simulink model "LAB_07_SIM_1"  (R2022b)
settings: Solver=ode4  StartTime=0.0  StopTime=10000  FixedStep=0.1  RelTol=1e-3
values from neighbouring files (symbols this model uses):
  a = 16371e+3    (= 16371000)    [lab_07_MAT.m]
  A0 = diag([1 1 1])    [LAB_04_17_OCT_MAT_KIN.m]    (also in LAB_05_24_OCT_MAT_KIN_COSDIR.m; LAB_06.m = A_target_fun(0); core_attitude_test.m = eye(3,3); lab_07_MAT.m)
  A_B1 = 2e-2    (= 0.02)    [lab_07_MAT.m]
  A_B2 = 6e-2    (= 0.06)    [lab_07_MAT.m]
  A_B3 = 2e-2    (= 0.02)    [lab_07_MAT.m]
  A_B4 = 6e-2    (= 0.06)    [lab_07_MAT.m]
  A_B5 = 3e-2    (= 0.03)    [lab_07_MAT.m]
  A_B6 = 3e-2    (= 0.03)    [lab_07_MAT.m]
  A_P1 = 12e-2    (= 0.12)    [lab_07_MAT.m]
  A_P2 = 12e-2    (= 0.12)    [lab_07_MAT.m]
  A_P3 = 12e-2    (= 0.12)    [lab_07_MAT.m]
  A_P4 = 12e-2    (= 0.12)    [lab_07_MAT.m]
  ang = deg2rad(11.5)    [lab_07_MAT.m]
  e = 0    [lab_07_MAT.m]
  g_1_0 = -29404.8    [lab_07_MAT.m]
  g_1_1 = -1450.9    [lab_07_MAT.m]
  h_1_1 = 4652.5    [lab_07_MAT.m]
  I = [Ix 0 0 ... (first row only)    [LAB_03_3_OCT_MAT_EUL_2_VERIFICATION.m]    (also in LAB_03_3_OCT_MAT_EUL_DOUBLESPIN.m = diag([Ix, Iy, Iz]); LAB_03_3_OCT_MAT_EUL_SPINAXIS.m = diag([Ix, Iy, Iz]); LAB_03_3_OCT_MAT_EUL_VECT.m; LAB_04_17_OCT_MAT_KIN.m)
  i = char('pippo')    [LAB_01_19_SEPT.m]    (also in lab_07_MAT.m = 0.1)
  j_B = [0.01; 0.05; 0.01]    [lab_07_MAT.m]
  N_B1 = [1,0,0]'    [lab_07_MAT.m]
  N_B2 = [0,1,0]'    [lab_07_MAT.m]
  N_B3 = [-1,0,0]'    [lab_07_MAT.m]
  N_B4 = [0,-1,0]'    [lab_07_MAT.m]
  N_B5 = [0,0,1]'    [lab_07_MAT.m]
  N_B6 = [0,0,-1]    [lab_07_MAT.m]
  N_P1 = [0,0,1]    [lab_07_MAT.m]
  N_P2 = [0,0,-1]    [lab_07_MAT.m]
  N_P3 = [0,0,1]    [lab_07_MAT.m]
  N_P4 = [0,0,-1]    [lab_07_MAT.m]
  n_rot = 0.0012    [lab_07_MAT.m]
  n_sun = 2*pi/T    (= 1.99238499086e-07)    [lab_07_MAT.m]
  om_0 = [om_x0, om_y0, om_z0]    [LAB_03_3_OCT_MAT_EUL.m]    (also in LAB_03_3_OCT_MAT_EUL_2_VERIFICATION.m = [om_x0; om_y0; om_z0]; LAB_03_3_OCT_MAT_EUL_DOUBLESPIN.m = [om_x0; om_y0; om_z0]; LAB_03_3_OCT_MAT_EUL_SPINAXIS.m = [om_x0; om_y0; om_z0]; LAB_03_3_OCT_MAT_EUL_VECT.m = [om_x0; om_y0; om_z0])
  P = [Px, Py, Pz]    [LAB_03_3_OCT_MAT_EUL_VECT.m]    (also in lab_07_MAT.m = 4.52666666667e-06)
  R = 6.371e+6 + H    (= 6381000)    [LAB_06.m]    (also in lab_07_MAT.m = 6378000)
  r_B1 = 1e-2*[15,0,0]    [lab_07_MAT.m]
  r_B2 = 1e-2*[0,5,0]    [lab_07_MAT.m]
  r_B3 = 1e-2*[-15,0,0]    [lab_07_MAT.m]
  r_B4 = 1e-2*[0,-5,0]    [lab_07_MAT.m]
  r_B5 = 1e-2*[0,0,10]    [lab_07_MAT.m]
  r_B6 = 1e-2*[0,0,-10]    [lab_07_MAT.m]
  r_P1 = 1e-2*[0,20,10]    [lab_07_MAT.m]
  r_P2 = 1e-2*[0,20,10]    [lab_07_MAT.m]
  r_P3 = 1e-2*[0,-20,10]    [lab_07_MAT.m]
  r_P4 = 1e-2*[0,-20,10]    [lab_07_MAT.m]
  r_sun = 149597870000    [lab_07_MAT.m]
  rho_d = 0.1    [lab_07_MAT.m]
  rho_sB = 0.5    [lab_07_MAT.m]
  rho_sP = 0.5    [lab_07_MAT.m]
  rot_E = 7.29e-5    (= 7.29e-05)    [lab_07_MAT.m]
  theta_0 = 3/2 * pi    (= 4.71238898038)    [lab_07_MAT.m]
libraries: matrix_library x12, sharedutil x1, vrlib x1
settings Model: Creator=maria  LastModifiedBy=maria

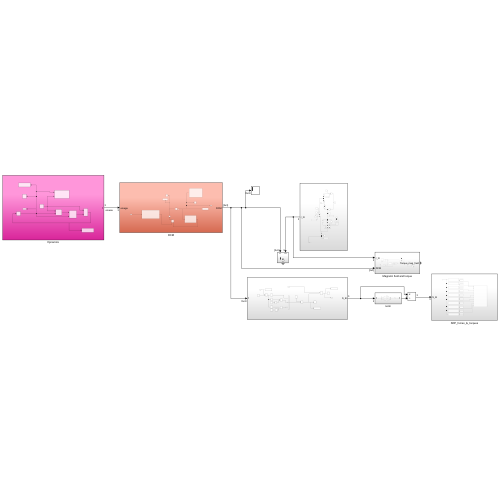
[thumbnail: Simulink's stored preview of the top-level diagram]
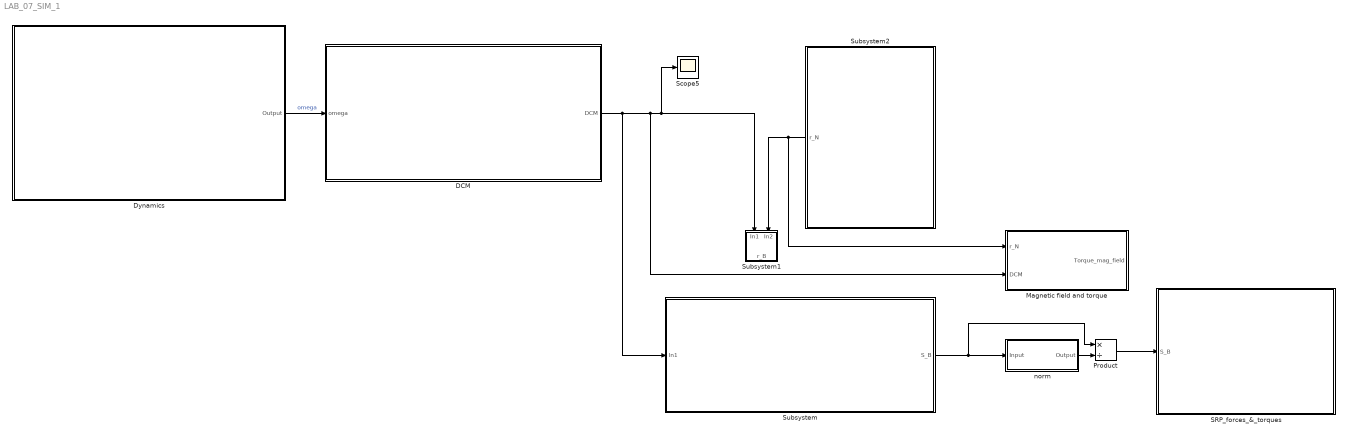
== system LAB_07_SIM_1 ==
  DCM : Subsystem
  Dynamics : Subsystem
  Magnetic field and torque : Subsystem
  Product : Product  Inputs=*/
  SRP_forces_&_torques : Subsystem
  Scope5 : Scope
  Subsystem : Subsystem
  Subsystem1 : Subsystem
  Subsystem2 : Subsystem
  norm : Subsystem
  wires:
  Dynamics/1(Output) -> DCM/1(omega)  "omega"
  DCM/1(DCM) -> Subsystem/1(In1), Magnetic field and torque/2(DCM), Subsystem1/1(In1), Scope5/1
  Subsystem2/1(r_N) -> Magnetic field and torque/1(r_N), Subsystem1/2(In2)
  Subsystem/1(S_B) -> Product/1, norm/1(Input)
  norm/1(Output) -> Product/2
  Product/1 -> SRP_forces_&_torques/1(S_B)

== system LAB_07_SIM_1/DCM ==
  note: A
  omega : Inport
  Determinant Chech fo Validation : Subsystem
  Gain1 : Gain  Gain=-1
  Integrator1 : Integrator  InitialCondition=A0
  Product2 : Product  Multiplication=Matrix(*)
  Scope1 : Scope
  Scope2 : Scope
  Subsystem : Subsystem
  To Workspace2 : ToWorkspace  VariableName=A  SampleTime=-1
  To Workspace3 : ToWorkspace  VariableName=A_dot  SampleTime=-1
  matrix of omega cross prod : Subsystem
  DCM : Outport
  wires:
  Integrator1/1 -> Subsystem/1(A1), Scope2/1, Determinant Chech fo Validation/1(DCM), DCM/1, To Workspace2/1
  matrix of omega cross prod/1(Out1) -> Product2/1
  Product2/1 -> Gain1/1  "A_dot"
  omega/1 -> matrix of omega cross prod/1(om)
  Gain1/1 -> Integrator1/1, To Workspace3/1, Scope1/1
  Subsystem/1(A_orthonormalized1) -> Product2/2

== system LAB_07_SIM_1/Dynamics ==
  Constant : Constant  Value=I
  Cross Product : matrix_library/Cross Product
  Integrator : Integrator  InitialCondition=om_0
  Product : Product  Multiplication=Matrix(*)
  Product1 : Product  Inputs=/*  Multiplication=Matrix(*)
  Scope : Scope
  To Workspace1 : ToWorkspace  VariableName=omega  SampleTime=-1
  To Workspace2 : ToWorkspace  VariableName=omega_dot  SampleTime=-1
  validation : Subsystem
  Output : Outport
  wires:
  Product1/1 -> To Workspace2/1, Integrator/1  "om_dot"
  Integrator/1 -> Product/2, Cross Product/2, validation/1(om), To Workspace1/1, Scope/1, Output/1  "om"
  Cross Product/1 -> Product1/2
  Constant/1 -> Product1/1, Product/1, validation/2(In2)  "I"
  Product/1 -> Cross Product/1

== system LAB_07_SIM_1/Magnetic field and torque ==
  r_N : Inport
  DCM : Inport  Port=2
  Constant : Constant  Value=j_B
  Constant10 : Constant  Value=3
  Constant5 : Constant  Value=R
  Constant9 : Constant  Value=3
  Cross Product : matrix_library/Cross Product
  Dot Product : DotProduct  OutDataTypeStr=Inherit: Inherit via internal rule
  Gain : Gain  Gain=1e-9
  Gain1 : Gain  Gain=3
  MatrixMultiply : Product  Multiplication=Matrix(*)
  Normalize Vector : vrlib/Utilities/Normalize Vector  maxzero=0
  Power : Math  Operator=pow
  Power1 : Math  Operator=pow
  Product3 : Product  Inputs=**/
  Product4 : Product
  Product5 : Product
  Scope : Scope
  Scope1 : Scope
  Scope3 : Scope
  Subsystem : Subsystem
  Sum1 : Sum  Inputs=-+
  To Workspace : ToWorkspace  VariableName=b_N  SampleTime=-1
  To Workspace3 : ToWorkspace  VariableName=Torque_mag_field  SampleTime=-1
  m : Subsystem
  norm1 : Subsystem
  Torque_mag_field : Outport
  wires:
  r_N/1 -> Normalize Vector/1, norm1/1(Input)
  Constant5/1 -> Power/1
  Constant9/1 -> Power/2
  Power/1 -> Product3/2
  Constant10/1 -> Power1/2
  norm1/1(Output) -> Power1/1  "r_norm"
  Power1/1 -> Product3/3
  Product3/1 -> Product4/1
  Dot Product/1 -> Product5/1
  m/1(m) -> Sum1/1, Dot Product/1
  Normalize Vector/1 -> Product5/2, Dot Product/2
  Product5/1 -> Gain1/1
  Sum1/1 -> Product4/2
  Subsystem/1(H0) -> Gain/1
  Product4/1 -> MatrixMultiply/2, To Workspace/1, Scope/1
  MatrixMultiply/1 -> Cross Product/2, Scope3/1, To Workspace3/1  "b_B"
  DCM/1 -> MatrixMultiply/1
  Constant/1 -> Cross Product/1
  Cross Product/1 -> Scope1/1, Torque_mag_field/1
  Gain1/1 -> Sum1/2
  Gain/1 -> Product3/1

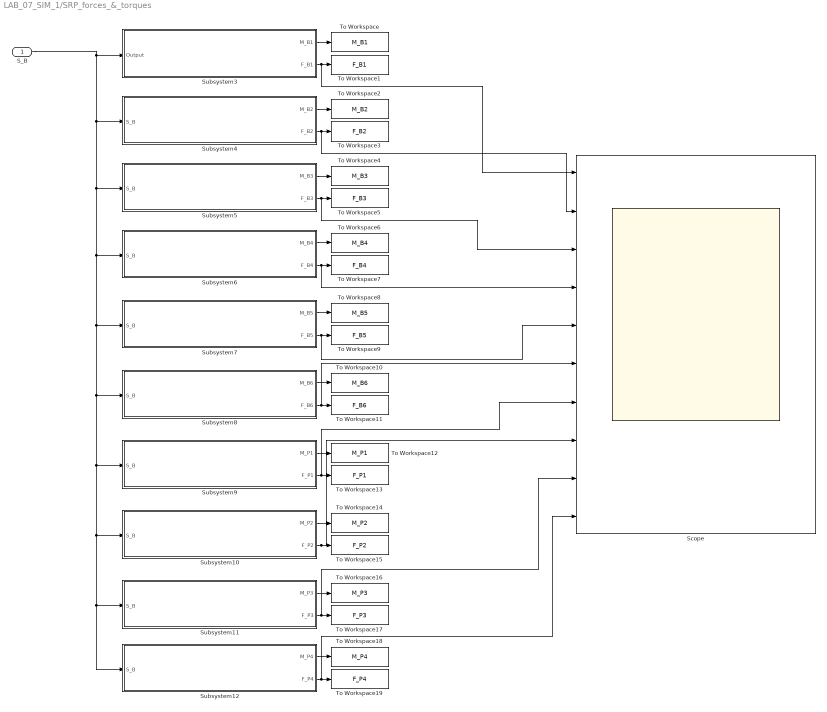
== system LAB_07_SIM_1/SRP_forces_&_torques ==
  S_B : Inport
  Scope : Scope  NumInputPorts=10
  Subsystem10 : Subsystem
  Subsystem11 : Subsystem
  Subsystem12 : Subsystem
  Subsystem3 : Subsystem
  Subsystem4 : Subsystem
  Subsystem5 : Subsystem
  Subsystem6 : Subsystem
  Subsystem7 : Subsystem
  Subsystem8 : Subsystem
  Subsystem9 : Subsystem
  To Workspace : ToWorkspace  VariableName=M_B1  SampleTime=-1
  To Workspace1 : ToWorkspace  VariableName=F_B1  SampleTime=-1
  To Workspace10 : ToWorkspace  VariableName=M_B6  SampleTime=-1
  To Workspace11 : ToWorkspace  VariableName=F_B6  SampleTime=-1
  To Workspace12 : ToWorkspace  VariableName=M_P1  SampleTime=-1
  To Workspace13 : ToWorkspace  VariableName=F_P1  SampleTime=-1
  To Workspace14 : ToWorkspace  VariableName=M_P2  SampleTime=-1
  To Workspace15 : ToWorkspace  VariableName=F_P2  SampleTime=-1
  To Workspace16 : ToWorkspace  VariableName=M_P3  SampleTime=-1
  To Workspace17 : ToWorkspace  VariableName=F_P3  SampleTime=-1
  To Workspace18 : ToWorkspace  VariableName=M_P4  SampleTime=-1
  To Workspace19 : ToWorkspace  VariableName=F_P4  SampleTime=-1
  To Workspace2 : ToWorkspace  VariableName=M_B2  SampleTime=-1
  To Workspace3 : ToWorkspace  VariableName=F_B2  SampleTime=-1
  To Workspace4 : ToWorkspace  VariableName=M_B3  SampleTime=-1
  To Workspace5 : ToWorkspace  VariableName=F_B3  SampleTime=-1
  To Workspace6 : ToWorkspace  VariableName=M_B4  SampleTime=-1
  To Workspace7 : ToWorkspace  VariableName=F_B4  SampleTime=-1
  To Workspace8 : ToWorkspace  VariableName=M_B5  SampleTime=-1
  To Workspace9 : ToWorkspace  VariableName=F_B5  SampleTime=-1
  wires:
  S_B/1 -> Subsystem11/1(S_B), Subsystem12/1(S_B), Subsystem10/1(S_B), Subsystem9/1(S_B), Subsystem8/1(S_B), Subsystem7/1(S_B), Subsystem6/1(S_B), Subsystem5/1(S_B), Subsystem4/1(S_B), Subsystem3/1(Output)
  Subsystem7/2(F_B5) -> Scope/5, To Workspace9/1
  Subsystem12/2(F_P4) -> Scope/10, To Workspace19/1
  Subsystem12/1(M_P4) -> To Workspace18/1
  Subsystem6/1(M_B4) -> To Workspace6/1
  Subsystem7/1(M_B5) -> To Workspace8/1
  Subsystem8/1(M_B6) -> To Workspace10/1
  Subsystem10/2(F_P2) -> Scope/8, To Workspace15/1
  Subsystem11/1(M_P3) -> To Workspace16/1
  Subsystem10/1(M_P2) -> To Workspace14/1
  Subsystem3/2(F_B1) -> Scope/1, To Workspace1/1
  Subsystem9/2(F_P1) -> Scope/7, To Workspace13/1
  Subsystem4/1(M_B2) -> To Workspace2/1
  Subsystem5/1(M_B3) -> To Workspace4/1
  Subsystem11/2(F_P3) -> Scope/9, To Workspace17/1
  Subsystem5/2(F_B3) -> Scope/3, To Workspace5/1
  Subsystem3/1(M_B1) -> To Workspace/1
  Subsystem8/2(F_B6) -> Scope/6, To Workspace11/1
  Subsystem6/2(F_B4) -> Scope/4, To Workspace7/1
  Subsystem4/2(F_B2) -> Scope/2, To Workspace3/1
  Subsystem9/1(M_P1) -> To Workspace12/1

== system LAB_07_SIM_1/Subsystem ==
  In1 : Inport
  Clock : Clock
  Constant6 : Constant  Value=n_sun
  Constant7 : Constant  Value=eps
  Constant8 : Constant  Value=eps
  Constant9 : Constant  Value=r_sun
  Cos4 : Trigonometry  Operator=cos
  Cos5 : Trigonometry  Operator=cos
  MatrixMultiply1 : Product  Multiplication=Matrix(*)
  Mux1 : Mux  Inputs=3
  Product{5..8} (4 alike) : Product
  Scope4 : Scope
  Scope6 : Scope
  Sin2 : Trigonometry
  Sin3 : Trigonometry
  Sin4 : Trigonometry
  To Workspace4 : ToWorkspace  VariableName=time  SampleTime=-1
  To Workspace5 : ToWorkspace  VariableName=simout1  SaveFormat=Timeseries  SampleTime=-1
  To Workspace6 : ToWorkspace  VariableName=S_B  SampleTime=-1
  S_B : Outport
  wires:
  Sin2/1 -> Product6/1
  Product8/1 -> MatrixMultiply1/2, To Workspace5/1, Scope4/1
  MatrixMultiply1/1 -> S_B/1, To Workspace6/1, Scope6/1  "S_B"
  Constant7/1 -> Cos5/1
  Constant8/1 -> Sin4/1
  Sin3/1 -> Product7/1
  In1/1 -> MatrixMultiply1/1
  Product7/1 -> Mux1/3
  Constant6/1 -> Product5/2
  Cos5/1 -> Product6/2
  Mux1/1 -> Product8/2
  Constant9/1 -> Product8/1
  Clock/1 -> Product5/1, To Workspace4/1
  Product5/1 -> Sin3/1, Sin2/1, Cos4/1
  Product6/1 -> Mux1/2
  Cos4/1 -> Mux1/1
  Sin4/1 -> Product7/2

== system LAB_07_SIM_1/Subsystem1 ==
  In1 : Inport
  In2 : Inport  Port=2
  MatrixMultiply : Product  Multiplication=Matrix(*)
  Scope3 : Scope
  To Workspace3 : ToWorkspace  VariableName=r_B  SampleTime=-1
  r_B : Outport
  wires:
  MatrixMultiply/1 -> r_B/1, To Workspace3/1, Scope3/1  "r_B"
  In2/1 -> MatrixMultiply/2
  In1/1 -> MatrixMultiply/1

== system LAB_07_SIM_1/Subsystem2 ==
  Constant : Constant
  Constant1 : Constant  Value=n_rot
  Constant2 : Constant  Value=(1-e^2)^(3/2)
  Constant3 : Constant  Value=a
  Constant4 : Constant  Value=(1-e^2)
  Constant5 : Constant  Value=i
  Cos : Trigonometry  Operator=cos
  Cos1 : Trigonometry  Operator=cos
  Cos2 : Trigonometry  Operator=cos
  Cos3 : Trigonometry
  Gain1 : Gain  Gain=e
  Integrator : Integrator  InitialCondition=theta_0  WrappedStateUpperValue=2*pi  WrappedStateLowerValue=0
  Mux : Mux  Inputs=3
  Product : Product  Inputs=**/
  Product1 : Product  Inputs=**/
  Product2 : Product
  Product3 : Product
  Product4 : Product
  Scope{,1..3} (4 alike) : Scope
  Sin : Trigonometry
  Sin1 : Trigonometry
  Square : Math  Operator=square
  Sum : Sum
  To Workspace : ToWorkspace  VariableName=r_N  SampleTime=-1
  To Workspace1 : ToWorkspace  VariableName=theta  SampleTime=-1
  To Workspace2 : ToWorkspace  VariableName=simout  SaveFormat=Timeseries  SampleTime=-1
  r_N : Outport
  wires:
  Product2/1 -> Mux/2
  Sin1/1 -> Product2/1
  Constant/1 -> Sum/1
  Integrator/1 -> Scope1/1, To Workspace1/1, Cos2/1, Sin1/1, Cos3/1, Cos/1  "theta"
  Product3/1 -> r_N/1, To Workspace/1, Scope/1
  Constant1/1 -> Product/1
  Sin/1 -> Product4/2
  Constant5/1 -> Cos1/1, Sin/1
  Cos3/1 -> Product4/1
  Constant3/1 -> Product1/1
  Square/1 -> Product/2
  Gain1/1 -> Sum/2
  Cos1/1 -> Product2/2
  Sum/1 -> Product1/3, Square/1
  Product/1 -> Scope3/1, Integrator/1  "theta_dot"
  Cos/1 -> Gain1/1
  Product4/1 -> Mux/3
  Cos2/1 -> Mux/1
  Mux/1 -> Product3/2  "r_N"
  Constant2/1 -> Product/3
  Product1/1 -> To Workspace2/1, Scope2/1, Product3/1  "r"
  Constant4/1 -> Product1/2

== system LAB_07_SIM_1/norm ==
  Input : Inport
  Demux : Demux  Outputs=3
  Sqrt : Sqrt
  Square : Math  Operator=square
  Square1 : Math  Operator=square
  Square2 : Math  Operator=square
  Sum : Sum  Inputs=+++
  Output : Outport
  wires:
  Square/1 -> Sum/1
  Square1/1 -> Sum/2
  Square2/1 -> Sum/3
  Sum/1 -> Sqrt/1
  Input/1 -> Demux/1
  Sqrt/1 -> Output/1
  Demux/1 -> Square/1
  Demux/2 -> Square1/1
  Demux/3 -> Square2/1

== system LAB_07_SIM_1/DCM/Determinant Chech fo Validation ==
  DCM : Inport
  Determinant of 3x3 Matrix : sharedutil/Determinant of 3x3 Matrix  aMode=aMode
      settings: LibrarySourceBlock=|
      | aerolibutil/Determinant of
      | 3x3 Matrix
  MATLAB Function : MATLAB Function  TreatAsAtomicUnit=on
  To Workspace : ToWorkspace  VariableName=perpendicularity_flag  SampleTime=-1
  To Workspace4 : ToWorkspace  VariableName=detA  SampleTime=-1
  determinant : Scope
  perpendicularity : Scope
  wires:
  Determinant of 3x3 Matrix/1 -> determinant/1, To Workspace4/1
  DCM/1 -> MATLAB Function/1(DCM), Determinant of 3x3 Matrix/1
  MATLAB Function/1(perpendicularity_flag) -> To Workspace/1, perpendicularity/1

== system LAB_07_SIM_1/DCM/Subsystem ==
  A1 : Inport
  Gain : Gain  Gain=1.5
  Gain1 : Gain  Gain=-0.5
  Gain4 : Gain  Commented=on  Gain=3/2
  Gain5 : Gain  Commented=on  Gain=1/2
  Product : Product  Inputs=3  Multiplication=Matrix(*)
  Product3 : Product  Commented=on  Inputs=3  Multiplication=Matrix(*)
  Sum : Sum  Commented=on  Inputs=+-
  Sum1 : Sum
  Transpose : Math  Commented=on  Operator=transpose
  Transpose1 : Math  Operator=transpose
  A_orthonormalized1 : Outport
  wires:
  Sum/1 -> ?
  Gain5/1 -> Sum/2
  Product3/1 -> Gain5/1
  Transpose/1 -> Product3/2  "A_transpose"
  Gain4/1 -> Sum/1
  A1/1 -> Product/1, Transpose1/1, Product/3, Gain/1
  Gain/1 -> Sum1/2
  Sum1/1 -> A_orthonormalized1/1
  Gain1/1 -> Sum1/1
  Product/1 -> Gain1/1
  Transpose1/1 -> Product/2

== system LAB_07_SIM_1/DCM/matrix of omega cross prod ==
  om : Inport
  Constant1 : Constant  Value=0
  Constant2 : Constant  Value=0
  Constant3 : Constant  Value=0
  Demux : Demux  Outputs=3
  Display : Display
  Gain : Gain  Gain=-1
  Gain1 : Gain  Gain=-1
  Gain2 : Gain  Gain=-1
  Matrix Concatenate : Concatenate  NumInputs=3  Mode=Multidimensional array
  Mux : Mux  Inputs=3
  Mux1 : Mux  Inputs=3
  Mux2 : Mux  Inputs=3
  Scope : Scope
  Selector : Selector  InputPortWidth=3  IndexOptions=Index vector (dialog)  Indices=[1 3]  OutputSizes=1
  Transpose : Math  Operator=transpose
  Transpose1 : Math  Operator=transpose
  Transpose2 : Math  Operator=transpose
  Out1 : Outport
  wires:
  Matrix Concatenate/1 -> Display/1, Scope/1, Out1/1
  Demux/1 -> Gain1/1, Mux2/2
  Mux1/1 -> Transpose1/1
  Constant3/1 -> Mux2/3
  Gain/1 -> Mux/2
  Gain2/1 -> Mux2/1
  Constant1/1 -> Mux/1
  Demux/3 -> Gain/1, Mux1/1
  Demux/2 -> Mux/3, Gain2/1
  Mux/1 -> Transpose/1
  Gain1/1 -> Mux1/3
  Mux2/1 -> Transpose2/1
  Constant2/1 -> Mux1/2
  om/1 -> Demux/1
  Transpose/1 -> Matrix Concatenate/1
  Transpose1/1 -> Matrix Concatenate/2
  Transpose2/1 -> Matrix Concatenate/3

== system LAB_07_SIM_1/Dynamics/validation ==
  om : Inport
  In2 : Inport  Port=2
  Gain : Gain  Gain=1/2
  Product : Product  Inputs=3  Multiplication=Matrix(*)
  Product2 : Product  Multiplication=Matrix(*)
  Scope : Scope
  Scope1 : Scope
  To Workspace : ToWorkspace  VariableName=E  SampleTime=-1
  To Workspace2 : ToWorkspace  VariableName=hnorm  SampleTime=-1
  Transpose1 : Math  Operator=transpose
  norm : Subsystem
  wires:
  Product2/1 -> norm/1(Input)
  norm/1(Output) -> To Workspace2/1, Scope1/1
  om/1 -> Transpose1/1, Product/3, Product2/2
  In2/1 -> Product/2, Product2/1  "I"
  Transpose1/1 -> Product/1
  Product/1 -> Gain/1
  Gain/1 -> Scope/1, To Workspace/1

== system LAB_07_SIM_1/Magnetic field and torque/Subsystem ==
  Constant6 : Constant  Value=g_1_0
  Constant7 : Constant  Value=g_1_1
  Constant8 : Constant  Value=h_1_1
  Sqrt : Sqrt
  Square : Math  Operator=square
  Square1 : Math  Operator=square
  Square2 : Math  Operator=square
  Sum : Sum  Inputs=+++
  H0 : Outport
  wires:
  Constant8/1 -> Square2/1
  Square2/1 -> Sum/3
  Constant6/1 -> Square/1
  Constant7/1 -> Square1/1
  Square/1 -> Sum/1
  Sum/1 -> Sqrt/1
  Sqrt/1 -> H0/1  "H0"
  Square1/1 -> Sum/2

== system LAB_07_SIM_1/Magnetic field and torque/m ==
  Clock : Clock
  Constant : Constant  Value=ang
  Constant2 : Constant  Value=rot_E
  Constant3 : Constant  Value=ang
  Constant4 : Constant  Value=ang
  Cos : Trigonometry  Operator=cos
  Cos1 : Trigonometry  Operator=cos
  Mux : Mux  Inputs=3
  Product : Product
  Product1 : Product
  Product2 : Product
  Scope : Scope
  Sin : Trigonometry
  Sin1 : Trigonometry
  Sin2 : Trigonometry
  norm : Subsystem
  m : Outport
  wires:
  Cos1/1 -> Product1/1
  Constant3/1 -> Sin1/1
  Product/1 -> Sin2/1, Cos1/1
  Constant/1 -> Sin/1
  Constant4/1 -> Cos/1
  Mux/1 -> m/1, norm/1(Input)  "m"
  Sin2/1 -> Product2/1
  Product2/1 -> Mux/2
  Constant2/1 -> Product/1
  Product1/1 -> Mux/1
  Sin1/1 -> Product2/2
  Clock/1 -> Product/2
  Sin/1 -> Product1/2
  Cos/1 -> Mux/3
  norm/1(Output) -> Scope/1

== system LAB_07_SIM_1/Magnetic field and torque/norm1 ==
  Input : Inport
  Demux : Demux  Outputs=3
  Sqrt : Sqrt
  Square : Math  Operator=square
  Square1 : Math  Operator=square
  Square2 : Math  Operator=square
  Sum : Sum  Inputs=+++
  Output : Outport
  wires:
  Square/1 -> Sum/1
  Square1/1 -> Sum/2
  Square2/1 -> Sum/3
  Sum/1 -> Sqrt/1
  Input/1 -> Demux/1
  Sqrt/1 -> Output/1
  Demux/1 -> Square/1
  Demux/2 -> Square1/1
  Demux/3 -> Square2/1

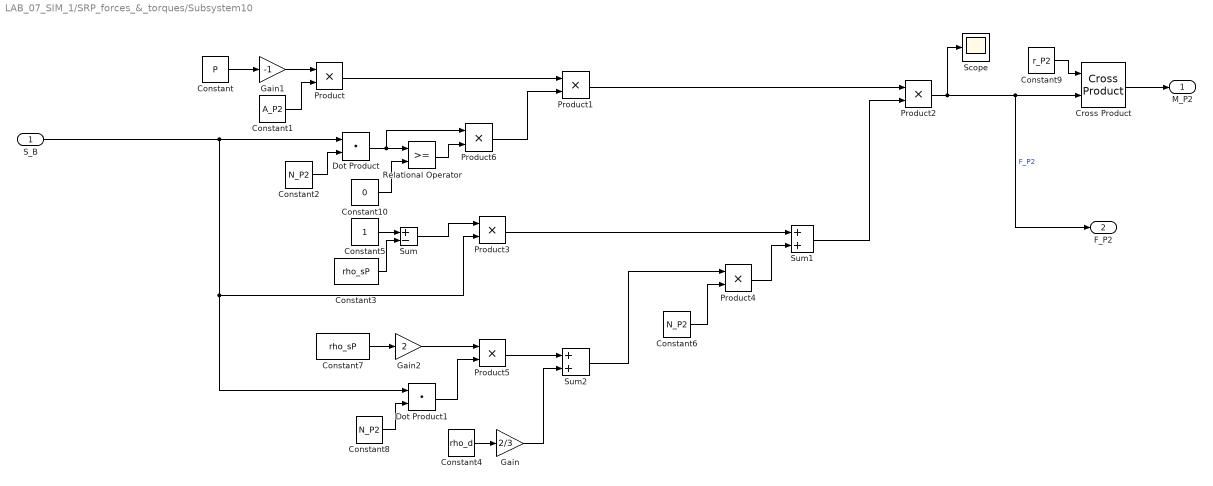
== system LAB_07_SIM_1/SRP_forces_&_torques/Subsystem10 ==
  S_B : Inport
  Constant : Constant  Value=P
  Constant1 : Constant  Value=A_P2
  Constant10 : Constant  Value=0
  Constant2 : Constant  Value=N_P2
  Constant3 : Constant  Value=rho_sP
  Constant4 : Constant  Value=rho_d
  Constant5 : Constant
  Constant6 : Constant  Value=N_P2
  Constant7 : Constant  Value=rho_sP
  Constant8 : Constant  Value=N_P2
  Constant9 : Constant  Value=r_P2
  Cross Product : matrix_library/Cross Product
  Dot Product : DotProduct  OutDataTypeStr=Inherit: Inherit via internal rule
  Dot Product1 : DotProduct  OutDataTypeStr=Inherit: Inherit via internal rule
  Gain : Gain  Gain=2/3
  Gain1 : Gain  Gain=-1
  Gain2 : Gain  Gain=2
  Product{,1..6} (7 alike) : Product
  Relational Operator : RelationalOperator  OutDataTypeStr=boolean  RndMeth=Simplest  InputSameDT=off
  Scope : Scope
  Sum : Sum  Inputs=+-
  Sum1 : Sum
  Sum2 : Sum
  M_P2 : Outport
  F_P2 : Outport  Port=2
  wires:
  Sum1/1 -> Product2/2
  Constant4/1 -> Gain/1
  Product/1 -> Product1/1
  Constant3/1 -> Sum/2
  Constant5/1 -> Sum/1
  Constant9/1 -> Cross Product/1
  Gain1/1 -> Product/1
  Dot Product1/1 -> Product5/2
  Product3/1 -> Sum1/1
  Cross Product/1 -> M_P2/1
  Constant1/1 -> Product/2
  Sum2/1 -> Product4/1
  Constant7/1 -> Gain2/1
  Constant/1 -> Gain1/1
  Gain2/1 -> Product5/1
  Gain/1 -> Sum2/2
  Constant2/1 -> Dot Product/2
  Product1/1 -> Product2/1
  Sum/1 -> Product3/1
  Constant6/1 -> Product4/2
  Constant8/1 -> Dot Product1/2
  Product4/1 -> Sum1/2
  Product5/1 -> Sum2/1
  Product2/1 -> Scope/1, Cross Product/2, F_P2/1  "F_P2"
  S_B/1 -> Product3/2, Dot Product1/1, Dot Product/1
  Constant10/1 -> Relational Operator/2
  Relational Operator/1 -> Product6/2
  Dot Product/1 -> Product6/1, Relational Operator/1
  Product6/1 -> Product1/2

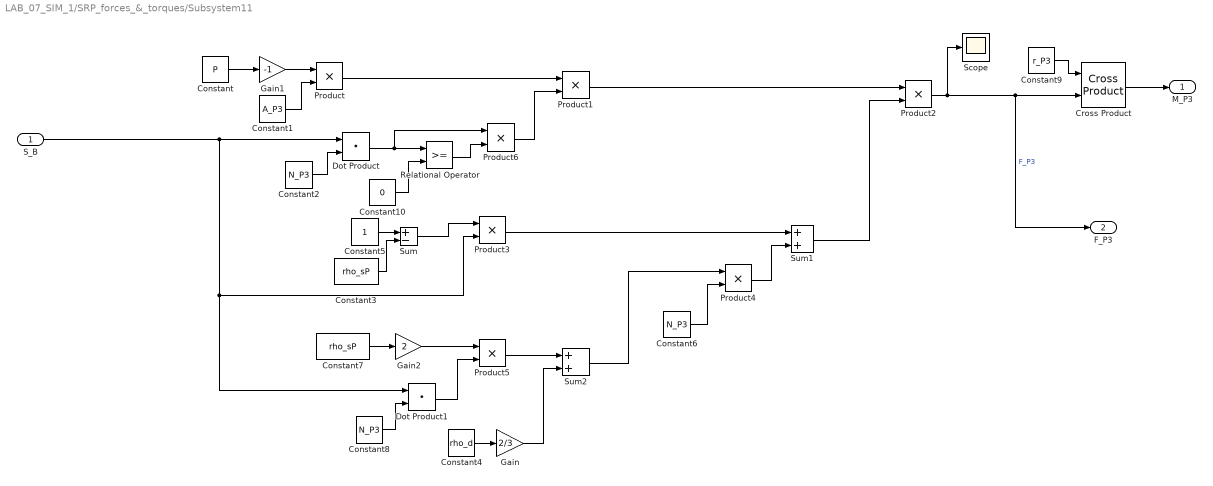
== system LAB_07_SIM_1/SRP_forces_&_torques/Subsystem11 ==
  S_B : Inport
  Constant : Constant  Value=P
  Constant1 : Constant  Value=A_P3
  Constant10 : Constant  Value=0
  Constant2 : Constant  Value=N_P3
  Constant3 : Constant  Value=rho_sP
  Constant4 : Constant  Value=rho_d
  Constant5 : Constant
  Constant6 : Constant  Value=N_P3
  Constant7 : Constant  Value=rho_sP
  Constant8 : Constant  Value=N_P3
  Constant9 : Constant  Value=r_P3
  Cross Product : matrix_library/Cross Product
  Dot Product : DotProduct  OutDataTypeStr=Inherit: Inherit via internal rule
  Dot Product1 : DotProduct  OutDataTypeStr=Inherit: Inherit via internal rule
  Gain : Gain  Gain=2/3
  Gain1 : Gain  Gain=-1
  Gain2 : Gain  Gain=2
  Product{,1..6} (7 alike) : Product
  Relational Operator : RelationalOperator  OutDataTypeStr=boolean  RndMeth=Simplest  InputSameDT=off
  Scope : Scope
  Sum : Sum  Inputs=+-
  Sum1 : Sum
  Sum2 : Sum
  M_P3 : Outport
  F_P3 : Outport  Port=2
  wires:
  S_B/1 -> Dot Product/1, Dot Product1/1, Product3/2
  Product2/1 -> F_P3/1, Cross Product/2, Scope/1  "F_P3"
  Product5/1 -> Sum2/1
  Product4/1 -> Sum1/2
  Constant8/1 -> Dot Product1/2
  Constant6/1 -> Product4/2
  Sum/1 -> Product3/1
  Product1/1 -> Product2/1
  Constant2/1 -> Dot Product/2
  Gain/1 -> Sum2/2
  Gain2/1 -> Product5/1
  Constant/1 -> Gain1/1
  Constant7/1 -> Gain2/1
  Sum2/1 -> Product4/1
  Constant1/1 -> Product/2
  Cross Product/1 -> M_P3/1
  Product3/1 -> Sum1/1
  Dot Product1/1 -> Product5/2
  Gain1/1 -> Product/1
  Constant9/1 -> Cross Product/1
  Constant5/1 -> Sum/1
  Constant3/1 -> Sum/2
  Product/1 -> Product1/1
  Constant4/1 -> Gain/1
  Sum1/1 -> Product2/2
  Constant10/1 -> Relational Operator/2
  Relational Operator/1 -> Product6/2
  Dot Product/1 -> Product6/1, Relational Operator/1
  Product6/1 -> Product1/2

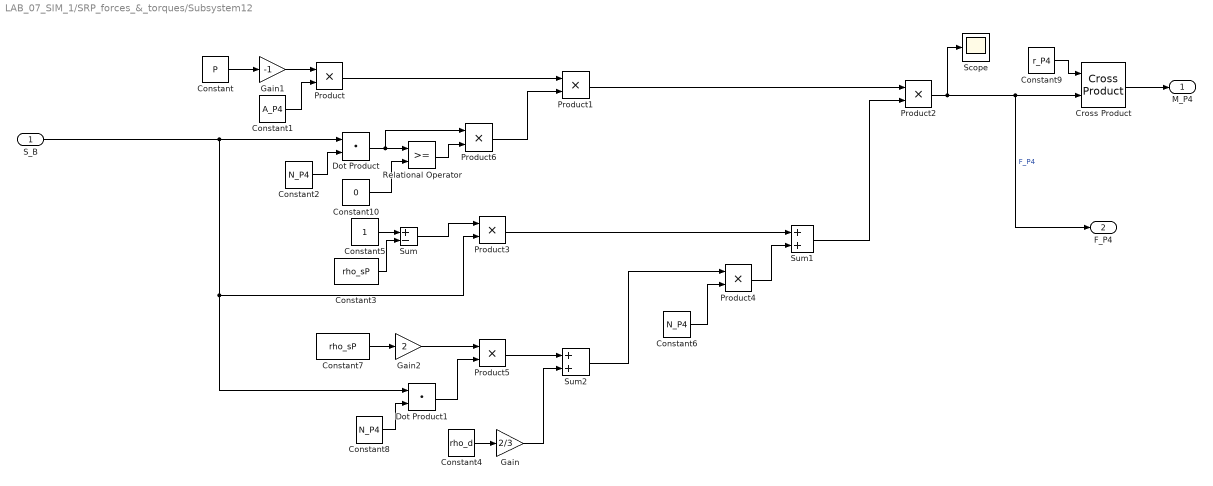
== system LAB_07_SIM_1/SRP_forces_&_torques/Subsystem12 ==
  S_B : Inport
  Constant : Constant  Value=P
  Constant1 : Constant  Value=A_P4
  Constant10 : Constant  Value=0
  Constant2 : Constant  Value=N_P4
  Constant3 : Constant  Value=rho_sP
  Constant4 : Constant  Value=rho_d
  Constant5 : Constant
  Constant6 : Constant  Value=N_P4
  Constant7 : Constant  Value=rho_sP
  Constant8 : Constant  Value=N_P4
  Constant9 : Constant  Value=r_P4
  Cross Product : matrix_library/Cross Product
  Dot Product : DotProduct  OutDataTypeStr=Inherit: Inherit via internal rule
  Dot Product1 : DotProduct  OutDataTypeStr=Inherit: Inherit via internal rule
  Gain : Gain  Gain=2/3
  Gain1 : Gain  Gain=-1
  Gain2 : Gain  Gain=2
  Product{,1..6} (7 alike) : Product
  Relational Operator : RelationalOperator  OutDataTypeStr=boolean  RndMeth=Simplest  InputSameDT=off
  Scope : Scope
  Sum : Sum  Inputs=+-
  Sum1 : Sum
  Sum2 : Sum
  M_P4 : Outport
  F_P4 : Outport  Port=2
  wires:
  Sum1/1 -> Product2/2
  Constant4/1 -> Gain/1
  Product/1 -> Product1/1
  Constant3/1 -> Sum/2
  Constant5/1 -> Sum/1
  Constant9/1 -> Cross Product/1
  Gain1/1 -> Product/1
  Dot Product1/1 -> Product5/2
  Product3/1 -> Sum1/1
  Cross Product/1 -> M_P4/1
  Constant1/1 -> Product/2
  Sum2/1 -> Product4/1
  Constant7/1 -> Gain2/1
  Constant/1 -> Gain1/1
  Gain2/1 -> Product5/1
  Gain/1 -> Sum2/2
  Constant2/1 -> Dot Product/2
  Product1/1 -> Product2/1
  Sum/1 -> Product3/1
  Constant6/1 -> Product4/2
  Constant8/1 -> Dot Product1/2
  Product4/1 -> Sum1/2
  Product5/1 -> Sum2/1
  Product2/1 -> Scope/1, Cross Product/2, F_P4/1  "F_P4"
  S_B/1 -> Product3/2, Dot Product1/1, Dot Product/1
  Constant10/1 -> Relational Operator/2
  Relational Operator/1 -> Product6/2
  Product6/1 -> Product1/2
  Dot Product/1 -> Product6/1, Relational Operator/1

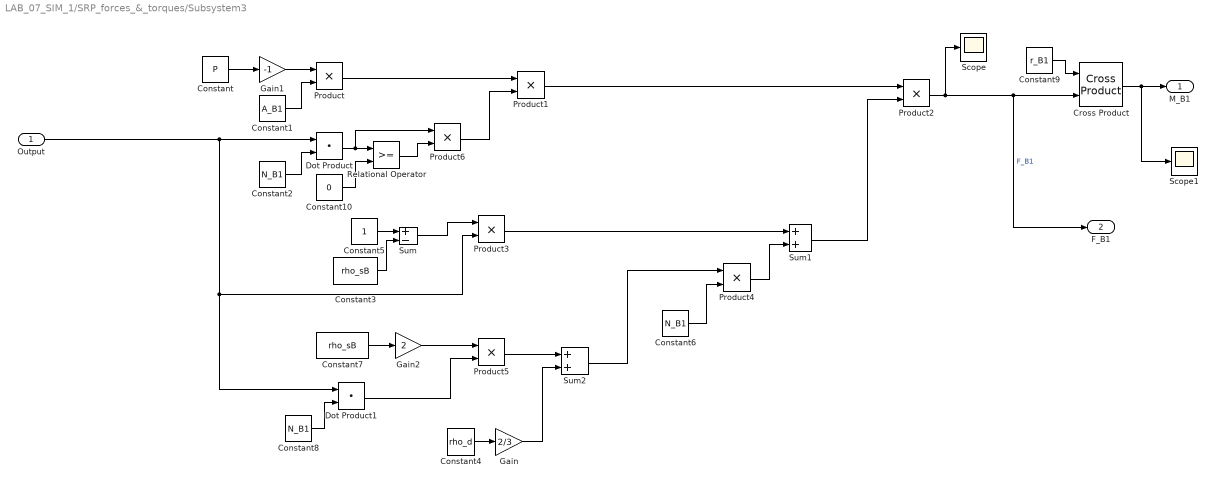
== system LAB_07_SIM_1/SRP_forces_&_torques/Subsystem3 ==
  Output : Inport
  Constant : Constant  Value=P
  Constant1 : Constant  Value=A_B1
  Constant10 : Constant  Value=0
  Constant2 : Constant  Value=N_B1
  Constant3 : Constant  Value=rho_sB
  Constant4 : Constant  Value=rho_d
  Constant5 : Constant
  Constant6 : Constant  Value=N_B1
  Constant7 : Constant  Value=rho_sB
  Constant8 : Constant  Value=N_B1
  Constant9 : Constant  Value=r_B1
  Cross Product : matrix_library/Cross Product
  Dot Product : DotProduct  OutDataTypeStr=Inherit: Inherit via internal rule
  Dot Product1 : DotProduct  OutDataTypeStr=Inherit: Inherit via internal rule
  Gain : Gain  Gain=2/3
  Gain1 : Gain  Gain=-1
  Gain2 : Gain  Gain=2
  Product{,1..6} (7 alike) : Product
  Relational Operator : RelationalOperator  OutDataTypeStr=boolean  RndMeth=Simplest  InputSameDT=off
  Scope : Scope
  Scope1 : Scope
  Sum : Sum  Inputs=+-
  Sum1 : Sum
  Sum2 : Sum
  M_B1 : Outport
  F_B1 : Outport  Port=2
  wires:
  Output/1 -> Dot Product/1, Dot Product1/1, Product3/2
  Product2/1 -> F_B1/1, Cross Product/2, Scope/1  "F_B1"
  Product5/1 -> Sum2/1
  Product4/1 -> Sum1/2
  Constant8/1 -> Dot Product1/2
  Constant6/1 -> Product4/2
  Sum/1 -> Product3/1
  Product1/1 -> Product2/1
  Constant2/1 -> Dot Product/2
  Gain/1 -> Sum2/2
  Gain2/1 -> Product5/1
  Constant/1 -> Gain1/1
  Constant7/1 -> Gain2/1
  Sum2/1 -> Product4/1
  Constant1/1 -> Product/2
  Cross Product/1 -> Scope1/1, M_B1/1
  Product3/1 -> Sum1/1
  Gain1/1 -> Product/1
  Constant9/1 -> Cross Product/1
  Constant5/1 -> Sum/1
  Constant3/1 -> Sum/2
  Product/1 -> Product1/1
  Constant4/1 -> Gain/1
  Sum1/1 -> Product2/2
  Constant10/1 -> Relational Operator/2
  Dot Product/1 -> Product6/1, Relational Operator/1
  Dot Product1/1 -> Product5/2
  Relational Operator/1 -> Product6/2
  Product6/1 -> Product1/2

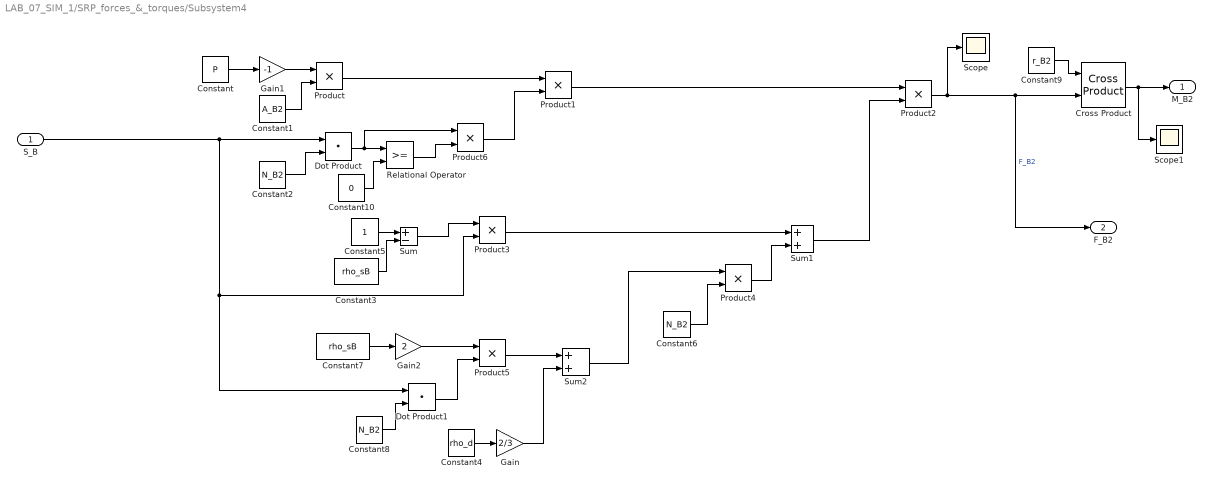
== system LAB_07_SIM_1/SRP_forces_&_torques/Subsystem4 ==
  S_B : Inport
  Constant : Constant  Value=P
  Constant1 : Constant  Value=A_B2
  Constant10 : Constant  Value=0
  Constant2 : Constant  Value=N_B2
  Constant3 : Constant  Value=rho_sB
  Constant4 : Constant  Value=rho_d
  Constant5 : Constant
  Constant6 : Constant  Value=N_B2
  Constant7 : Constant  Value=rho_sB
  Constant8 : Constant  Value=N_B2
  Constant9 : Constant  Value=r_B2
  Cross Product : matrix_library/Cross Product
  Dot Product : DotProduct  OutDataTypeStr=Inherit: Inherit via internal rule
  Dot Product1 : DotProduct  OutDataTypeStr=Inherit: Inherit via internal rule
  Gain : Gain  Gain=2/3
  Gain1 : Gain  Gain=-1
  Gain2 : Gain  Gain=2
  Product{,1..6} (7 alike) : Product
  Relational Operator : RelationalOperator  OutDataTypeStr=boolean  RndMeth=Simplest  InputSameDT=off
  Scope : Scope
  Scope1 : Scope
  Sum : Sum  Inputs=+-
  Sum1 : Sum
  Sum2 : Sum
  M_B2 : Outport
  F_B2 : Outport  Port=2
  wires:
  Sum1/1 -> Product2/2
  Constant4/1 -> Gain/1
  Product/1 -> Product1/1
  Constant3/1 -> Sum/2
  Constant5/1 -> Sum/1
  Constant9/1 -> Cross Product/1
  Gain1/1 -> Product/1
  Dot Product1/1 -> Product5/2
  Product3/1 -> Sum1/1
  Cross Product/1 -> Scope1/1, M_B2/1
  Constant1/1 -> Product/2
  Sum2/1 -> Product4/1
  Constant7/1 -> Gain2/1
  Constant/1 -> Gain1/1
  Gain2/1 -> Product5/1
  Gain/1 -> Sum2/2
  Constant2/1 -> Dot Product/2
  Product1/1 -> Product2/1
  Sum/1 -> Product3/1
  Constant6/1 -> Product4/2
  Constant8/1 -> Dot Product1/2
  Product4/1 -> Sum1/2
  Product5/1 -> Sum2/1
  Product2/1 -> Scope/1, Cross Product/2, F_B2/1  "F_B2"
  S_B/1 -> Product3/2, Dot Product1/1, Dot Product/1
  Dot Product/1 -> Product6/1, Relational Operator/1
  Constant10/1 -> Relational Operator/2
  Relational Operator/1 -> Product6/2
  Product6/1 -> Product1/2

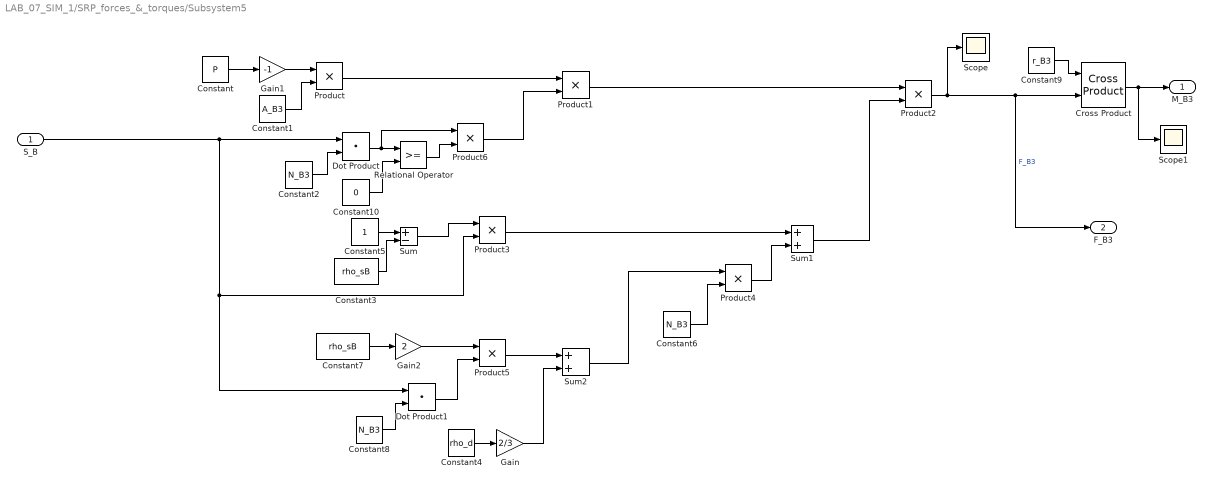
== system LAB_07_SIM_1/SRP_forces_&_torques/Subsystem5 ==
  S_B : Inport
  Constant : Constant  Value=P
  Constant1 : Constant  Value=A_B3
  Constant10 : Constant  Value=0
  Constant2 : Constant  Value=N_B3
  Constant3 : Constant  Value=rho_sB
  Constant4 : Constant  Value=rho_d
  Constant5 : Constant
  Constant6 : Constant  Value=N_B3
  Constant7 : Constant  Value=rho_sB
  Constant8 : Constant  Value=N_B3
  Constant9 : Constant  Value=r_B3
  Cross Product : matrix_library/Cross Product
  Dot Product : DotProduct  OutDataTypeStr=Inherit: Inherit via internal rule
  Dot Product1 : DotProduct  OutDataTypeStr=Inherit: Inherit via internal rule
  Gain : Gain  Gain=2/3
  Gain1 : Gain  Gain=-1
  Gain2 : Gain  Gain=2
  Product{,1..6} (7 alike) : Product
  Relational Operator : RelationalOperator  OutDataTypeStr=boolean  RndMeth=Simplest  InputSameDT=off
  Scope : Scope
  Scope1 : Scope
  Sum : Sum  Inputs=+-
  Sum1 : Sum
  Sum2 : Sum
  M_B3 : Outport
  F_B3 : Outport  Port=2
  wires:
  S_B/1 -> Dot Product/1, Dot Product1/1, Product3/2
  Product2/1 -> F_B3/1, Cross Product/2, Scope/1  "F_B3"
  Product5/1 -> Sum2/1
  Product4/1 -> Sum1/2
  Constant8/1 -> Dot Product1/2
  Constant6/1 -> Product4/2
  Sum/1 -> Product3/1
  Product1/1 -> Product2/1
  Constant2/1 -> Dot Product/2
  Gain/1 -> Sum2/2
  Gain2/1 -> Product5/1
  Constant/1 -> Gain1/1
  Constant7/1 -> Gain2/1
  Sum2/1 -> Product4/1
  Constant1/1 -> Product/2
  Cross Product/1 -> Scope1/1, M_B3/1
  Product3/1 -> Sum1/1
  Dot Product1/1 -> Product5/2
  Gain1/1 -> Product/1
  Constant9/1 -> Cross Product/1
  Constant5/1 -> Sum/1
  Constant3/1 -> Sum/2
  Product/1 -> Product1/1
  Constant4/1 -> Gain/1
  Sum1/1 -> Product2/2
  Constant10/1 -> Relational Operator/2
  Relational Operator/1 -> Product6/2
  Product6/1 -> Product1/2
  Dot Product/1 -> Product6/1, Relational Operator/1

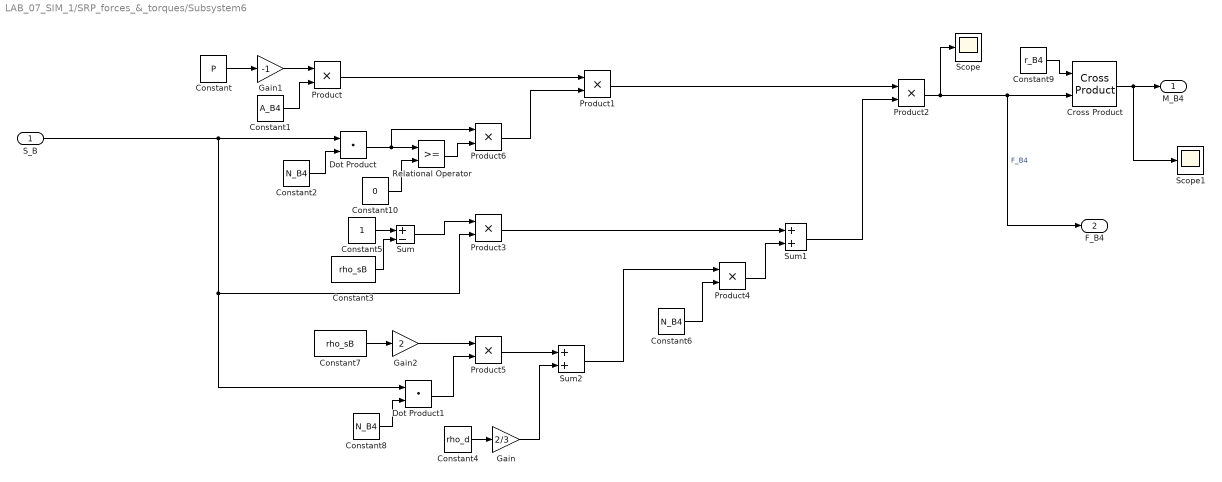
== system LAB_07_SIM_1/SRP_forces_&_torques/Subsystem6 ==
  S_B : Inport
  Constant : Constant  Value=P
  Constant1 : Constant  Value=A_B4
  Constant10 : Constant  Value=0
  Constant2 : Constant  Value=N_B4
  Constant3 : Constant  Value=rho_sB
  Constant4 : Constant  Value=rho_d
  Constant5 : Constant
  Constant6 : Constant  Value=N_B4
  Constant7 : Constant  Value=rho_sB
  Constant8 : Constant  Value=N_B4
  Constant9 : Constant  Value=r_B4
  Cross Product : matrix_library/Cross Product
  Dot Product : DotProduct  OutDataTypeStr=Inherit: Inherit via internal rule
  Dot Product1 : DotProduct  OutDataTypeStr=Inherit: Inherit via internal rule
  Gain : Gain  Gain=2/3
  Gain1 : Gain  Gain=-1
  Gain2 : Gain  Gain=2
  Product{,1..6} (7 alike) : Product
  Relational Operator : RelationalOperator  OutDataTypeStr=boolean  RndMeth=Simplest  InputSameDT=off
  Scope : Scope
  Scope1 : Scope
  Sum : Sum  Inputs=+-
  Sum1 : Sum
  Sum2 : Sum
  M_B4 : Outport
  F_B4 : Outport  Port=2
  wires:
  Sum1/1 -> Product2/2
  Constant4/1 -> Gain/1
  Product/1 -> Product1/1
  Constant3/1 -> Sum/2
  Constant5/1 -> Sum/1
  Constant9/1 -> Cross Product/1
  Gain1/1 -> Product/1
  Dot Product1/1 -> Product5/2
  Product3/1 -> Sum1/1
  Cross Product/1 -> Scope1/1, M_B4/1
  Constant1/1 -> Product/2
  Sum2/1 -> Product4/1
  Constant7/1 -> Gain2/1
  Constant/1 -> Gain1/1
  Gain2/1 -> Product5/1
  Gain/1 -> Sum2/2
  Constant2/1 -> Dot Product/2
  Product1/1 -> Product2/1
  Sum/1 -> Product3/1
  Constant6/1 -> Product4/2
  Constant8/1 -> Dot Product1/2
  Product4/1 -> Sum1/2
  Product5/1 -> Sum2/1
  Product2/1 -> Scope/1, Cross Product/2, F_B4/1  "F_B4"
  S_B/1 -> Product3/2, Dot Product1/1, Dot Product/1
  Constant10/1 -> Relational Operator/2
  Relational Operator/1 -> Product6/2
  Product6/1 -> Product1/2
  Dot Product/1 -> Product6/1, Relational Operator/1

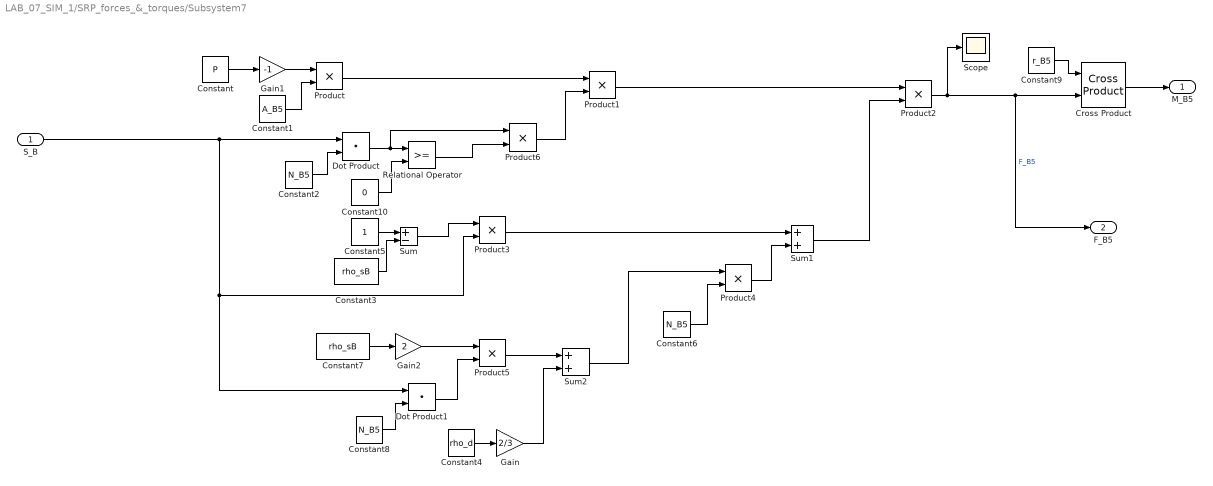
== system LAB_07_SIM_1/SRP_forces_&_torques/Subsystem7 ==
  S_B : Inport
  Constant : Constant  Value=P
  Constant1 : Constant  Value=A_B5
  Constant10 : Constant  Value=0
  Constant2 : Constant  Value=N_B5
  Constant3 : Constant  Value=rho_sB
  Constant4 : Constant  Value=rho_d
  Constant5 : Constant
  Constant6 : Constant  Value=N_B5
  Constant7 : Constant  Value=rho_sB
  Constant8 : Constant  Value=N_B5
  Constant9 : Constant  Value=r_B5
  Cross Product : matrix_library/Cross Product
  Dot Product : DotProduct  OutDataTypeStr=Inherit: Inherit via internal rule
  Dot Product1 : DotProduct  OutDataTypeStr=Inherit: Inherit via internal rule
  Gain : Gain  Gain=2/3
  Gain1 : Gain  Gain=-1
  Gain2 : Gain  Gain=2
  Product{,1..6} (7 alike) : Product
  Relational Operator : RelationalOperator  OutDataTypeStr=boolean  RndMeth=Simplest  InputSameDT=off
  Scope : Scope
  Sum : Sum  Inputs=+-
  Sum1 : Sum
  Sum2 : Sum
  M_B5 : Outport
  F_B5 : Outport  Port=2
  wires:
  S_B/1 -> Dot Product/1, Dot Product1/1, Product3/2
  Product2/1 -> F_B5/1, Cross Product/2, Scope/1  "F_B5"
  Product5/1 -> Sum2/1
  Product4/1 -> Sum1/2
  Constant8/1 -> Dot Product1/2
  Constant6/1 -> Product4/2
  Sum/1 -> Product3/1
  Product1/1 -> Product2/1
  Constant2/1 -> Dot Product/2
  Gain/1 -> Sum2/2
  Gain2/1 -> Product5/1
  Constant/1 -> Gain1/1
  Constant7/1 -> Gain2/1
  Sum2/1 -> Product4/1
  Constant1/1 -> Product/2
  Cross Product/1 -> M_B5/1
  Product3/1 -> Sum1/1
  Dot Product1/1 -> Product5/2
  Gain1/1 -> Product/1
  Constant9/1 -> Cross Product/1
  Constant5/1 -> Sum/1
  Constant3/1 -> Sum/2
  Product/1 -> Product1/1
  Constant4/1 -> Gain/1
  Sum1/1 -> Product2/2
  Constant10/1 -> Relational Operator/2
  Relational Operator/1 -> Product6/2
  Product6/1 -> Product1/2
  Dot Product/1 -> Product6/1, Relational Operator/1

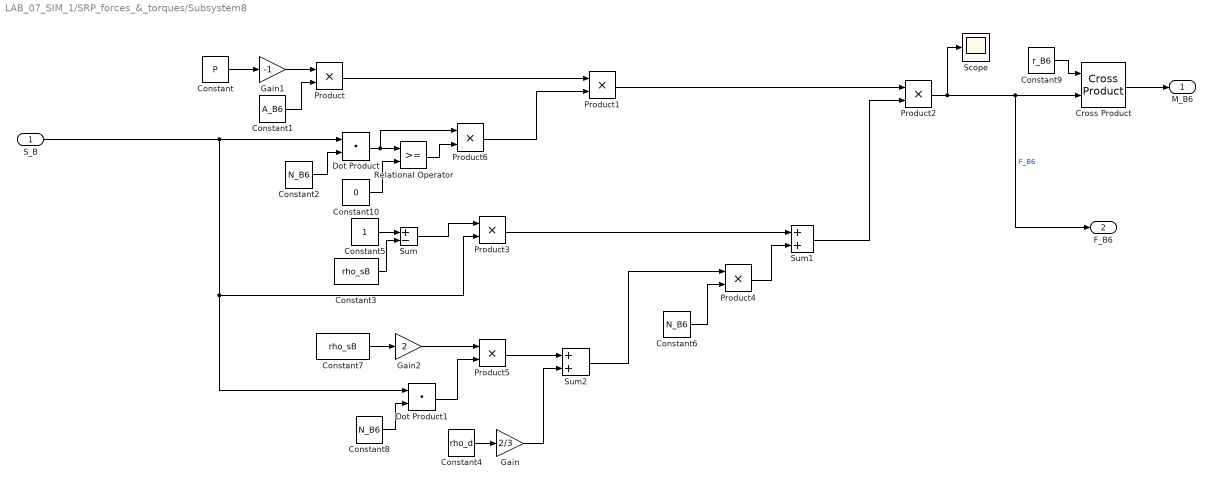
== system LAB_07_SIM_1/SRP_forces_&_torques/Subsystem8 ==
  S_B : Inport
  Constant : Constant  Value=P
  Constant1 : Constant  Value=A_B6
  Constant10 : Constant  Value=0
  Constant2 : Constant  Value=N_B6
  Constant3 : Constant  Value=rho_sB
  Constant4 : Constant  Value=rho_d
  Constant5 : Constant
  Constant6 : Constant  Value=N_B6
  Constant7 : Constant  Value=rho_sB
  Constant8 : Constant  Value=N_B6
  Constant9 : Constant  Value=r_B6
  Cross Product : matrix_library/Cross Product
  Dot Product : DotProduct  OutDataTypeStr=Inherit: Inherit via internal rule
  Dot Product1 : DotProduct  OutDataTypeStr=Inherit: Inherit via internal rule
  Gain : Gain  Gain=2/3
  Gain1 : Gain  Gain=-1
  Gain2 : Gain  Gain=2
  Product{,1..6} (7 alike) : Product
  Relational Operator : RelationalOperator  OutDataTypeStr=boolean  RndMeth=Simplest  InputSameDT=off
  Scope : Scope
  Sum : Sum  Inputs=+-
  Sum1 : Sum
  Sum2 : Sum
  M_B6 : Outport
  F_B6 : Outport  Port=2
  wires:
  Sum1/1 -> Product2/2
  Constant4/1 -> Gain/1
  Product/1 -> Product1/1
  Constant3/1 -> Sum/2
  Constant5/1 -> Sum/1
  Constant9/1 -> Cross Product/1
  Gain1/1 -> Product/1
  Dot Product1/1 -> Product5/2
  Product3/1 -> Sum1/1
  Cross Product/1 -> M_B6/1
  Constant1/1 -> Product/2
  Sum2/1 -> Product4/1
  Constant7/1 -> Gain2/1
  Constant/1 -> Gain1/1
  Gain2/1 -> Product5/1
  Gain/1 -> Sum2/2
  Constant2/1 -> Dot Product/2
  Product1/1 -> Product2/1
  Sum/1 -> Product3/1
  Constant6/1 -> Product4/2
  Constant8/1 -> Dot Product1/2
  Product4/1 -> Sum1/2
  Product5/1 -> Sum2/1
  Product2/1 -> Scope/1, Cross Product/2, F_B6/1  "F_B6"
  S_B/1 -> Product3/2, Dot Product1/1, Dot Product/1
  Constant10/1 -> Relational Operator/2
  Relational Operator/1 -> Product6/2
  Product6/1 -> Product1/2
  Dot Product/1 -> Product6/1, Relational Operator/1

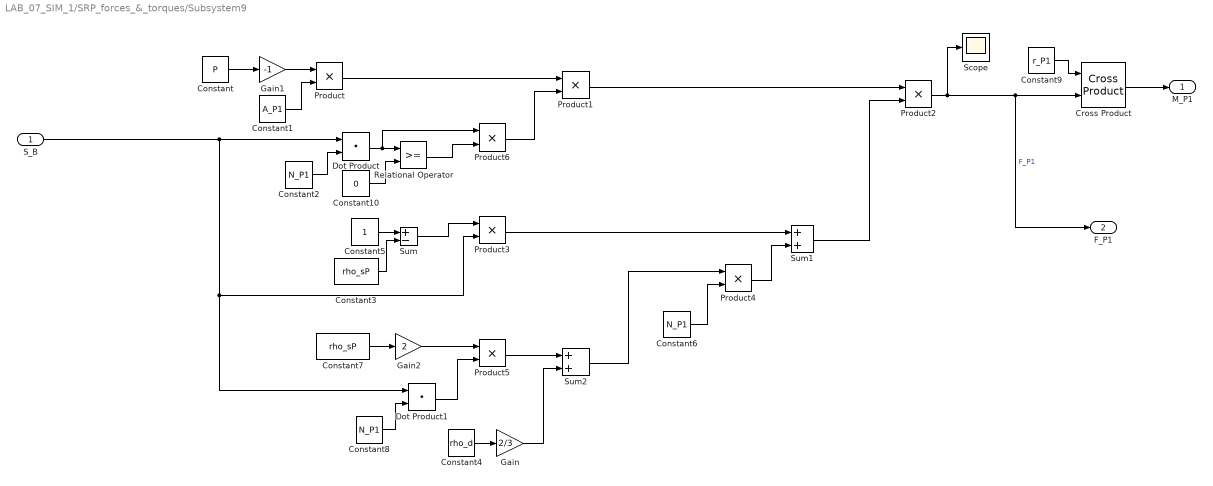
== system LAB_07_SIM_1/SRP_forces_&_torques/Subsystem9 ==
  S_B : Inport
  Constant : Constant  Value=P
  Constant1 : Constant  Value=A_P1
  Constant10 : Constant  Value=0
  Constant2 : Constant  Value=N_P1
  Constant3 : Constant  Value=rho_sP
  Constant4 : Constant  Value=rho_d
  Constant5 : Constant
  Constant6 : Constant  Value=N_P1
  Constant7 : Constant  Value=rho_sP
  Constant8 : Constant  Value=N_P1
  Constant9 : Constant  Value=r_P1
  Cross Product : matrix_library/Cross Product
  Dot Product : DotProduct  OutDataTypeStr=Inherit: Inherit via internal rule
  Dot Product1 : DotProduct  OutDataTypeStr=Inherit: Inherit via internal rule
  Gain : Gain  Gain=2/3
  Gain1 : Gain  Gain=-1
  Gain2 : Gain  Gain=2
  Product{,1..6} (7 alike) : Product
  Relational Operator : RelationalOperator  OutDataTypeStr=boolean  RndMeth=Simplest  InputSameDT=off
  Scope : Scope
  Sum : Sum  Inputs=+-
  Sum1 : Sum
  Sum2 : Sum
  M_P1 : Outport
  F_P1 : Outport  Port=2
  wires:
  S_B/1 -> Dot Product/1, Dot Product1/1, Product3/2
  Product2/1 -> F_P1/1, Cross Product/2, Scope/1  "F_P1"
  Product5/1 -> Sum2/1
  Product4/1 -> Sum1/2
  Constant8/1 -> Dot Product1/2
  Constant6/1 -> Product4/2
  Sum/1 -> Product3/1
  Product1/1 -> Product2/1
  Constant2/1 -> Dot Product/2
  Gain/1 -> Sum2/2
  Gain2/1 -> Product5/1
  Constant/1 -> Gain1/1
  Constant7/1 -> Gain2/1
  Sum2/1 -> Product4/1
  Constant1/1 -> Product/2
  Cross Product/1 -> M_P1/1
  Product3/1 -> Sum1/1
  Dot Product1/1 -> Product5/2
  Gain1/1 -> Product/1
  Constant9/1 -> Cross Product/1
  Constant5/1 -> Sum/1
  Constant3/1 -> Sum/2
  Product/1 -> Product1/1
  Constant4/1 -> Gain/1
  Sum1/1 -> Product2/2
  Constant10/1 -> Relational Operator/2
  Relational Operator/1 -> Product6/2
  Product6/1 -> Product1/2
  Dot Product/1 -> Product6/1, Relational Operator/1

== system LAB_07_SIM_1/Dynamics/validation/norm ==
  Input : Inport
  Demux : Demux  Outputs=3
  Sqrt : Sqrt
  Square : Math  Operator=square
  Square1 : Math  Operator=square
  Square2 : Math  Operator=square
  Sum : Sum  Inputs=+++
  Output : Outport
  wires:
  Square/1 -> Sum/1
  Square1/1 -> Sum/2
  Square2/1 -> Sum/3
  Sum/1 -> Sqrt/1
  Input/1 -> Demux/1
  Sqrt/1 -> Output/1
  Demux/1 -> Square/1
  Demux/2 -> Square1/1
  Demux/3 -> Square2/1

== system LAB_07_SIM_1/Magnetic field and torque/m/norm ==
  Input : Inport
  Demux : Demux  Outputs=3
  Sqrt : Sqrt
  Square : Math  Operator=square
  Square1 : Math  Operator=square
  Square2 : Math  Operator=square
  Sum : Sum  Inputs=+++
  Output : Outport
  wires:
  Square/1 -> Sum/1
  Square1/1 -> Sum/2
  Square2/1 -> Sum/3
  Sum/1 -> Sqrt/1
  Input/1 -> Demux/1
  Sqrt/1 -> Output/1
  Demux/1 -> Square/1
  Demux/2 -> Square1/1
  Demux/3 -> Square2/1

== matlab function LAB_07_SIM_1/DCM/Determinant Chech fo Validation/MATLAB Function ==
  data: DCM input; perpendicularity_flag output
function perpendicularity_flag = fcn(DCM)


perpendicularity_flag =zeros(3,1);

    x   = DCM(1,:);
    y   = DCM(2,:);
    z   = DCM(3,:);

    perpendicularity_flag(1)=dot(x,y);
    perpendicularity_flag(2)=dot(x,z);
    perpendicularity_flag(3)=dot(z,y);

end
